simulink model "solar_power_grid"  (R2026a)
settings: Solver=ode45  StopTime=20.0  MaxStep=0.01
libraries: simulink x1
settings Model: Creator=sanmaestro7  LastModifiedBy=sanmaestro7

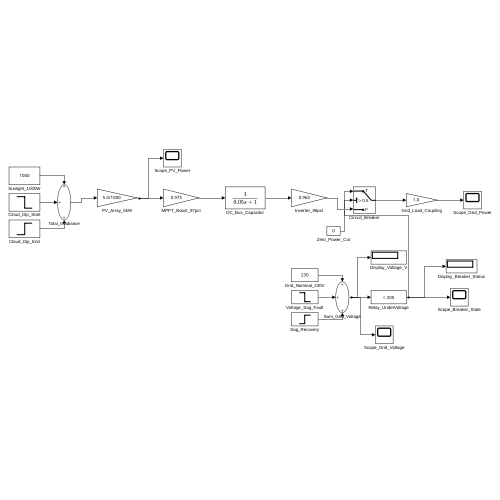
[thumbnail: Simulink's stored preview of the top-level diagram]
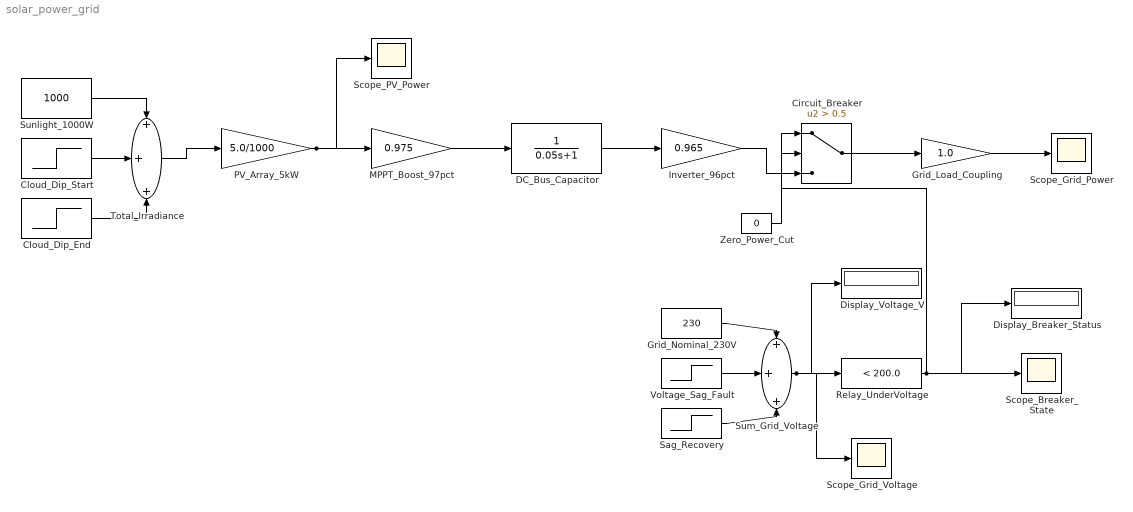
== system solar_power_grid ==
  Circuit_Breaker : Switch  Criteria=u2 > Threshold  Threshold=0.5  SaturateOnIntegerOverflow=off  InputSameDT=off
  Cloud_Dip_End : Step  Time=9  FinalValue=450  SampleTime=0
  Cloud_Dip_Start : Step  Time=5  FinalValue=-450  SampleTime=0
  DC_Bus_Capacitor : TransferFcn  Denominator=[0.05 1]
  Display_Breaker_Status : Display
  Display_Voltage_V : Display
  Grid_Load_Coupling : Gain  Gain=1.0
  Grid_Nominal_230V : Constant  Value=230
  Inverter_96pct : Gain  Gain=0.965
  MPPT_Boost_97pct : Gain  Gain=0.975
  PV_Array_5kW : Gain  Gain=5.0/1000
  Relay_UnderVoltage : simulink/Logic and Bit Operations/Compare To Constant  relop=<  const=200.0  OutDataTypeStr=boolean
  Sag_Recovery : Step  Time=15  FinalValue=46  SampleTime=0
  Scope_Breaker_State : Scope
  Scope_Grid_Power : Scope
  Scope_Grid_Voltage : Scope
  Scope_PV_Power : Scope
  Sum_Grid_Voltage : Sum  Inputs=+++
  Sunlight_1000W : Constant  Value=1000
  Total_Irradiance : Sum  Inputs=+++
  Voltage_Sag_Fault : Step  Time=12  FinalValue=-46  SampleTime=0
  Zero_Power_Cut : Constant  Value=0
  wires:
  Sunlight_1000W/1 -> Total_Irradiance/1
  Cloud_Dip_Start/1 -> Total_Irradiance/2
  Cloud_Dip_End/1 -> Total_Irradiance/3
  Total_Irradiance/1 -> PV_Array_5kW/1
  PV_Array_5kW/1 -> MPPT_Boost_97pct/1, Scope_PV_Power/1
  MPPT_Boost_97pct/1 -> DC_Bus_Capacitor/1
  DC_Bus_Capacitor/1 -> Inverter_96pct/1
  Inverter_96pct/1 -> Circuit_Breaker/3
  Zero_Power_Cut/1 -> Circuit_Breaker/1
  Circuit_Breaker/1 -> Grid_Load_Coupling/1
  Grid_Load_Coupling/1 -> Scope_Grid_Power/1
  Grid_Nominal_230V/1 -> Sum_Grid_Voltage/1
  Voltage_Sag_Fault/1 -> Sum_Grid_Voltage/2
  Sag_Recovery/1 -> Sum_Grid_Voltage/3
  Sum_Grid_Voltage/1 -> Relay_UnderVoltage/1, Scope_Grid_Voltage/1, Display_Voltage_V/1
  Relay_UnderVoltage/1 -> Circuit_Breaker/2, Scope_Breaker_State/1, Display_Breaker_Status/1
